simulink model "tanksReal"  (R2023a)
settings: Solver=VariableStepAuto  StartTime=0.0  StopTime=150  RelTol=1e-3
values from neighbouring files (symbols this model uses):
  a1 = 0.145    [main.m]
  a2 = 0.150    (= 0.15)    [main.m]
  A_a = 35    [main.m]
  fh = [3 4 5 6 7 8 9 10 11 12 13 14 15]    [main.m]
  fq = [17.75 21.65 23.76 27.55 30.01 31.98 33.88 38.18 46.28 49.88]    [main.m]
  fu = [0.5 1 1.5 2 2.5 3 3.5 5 8 10]    [main.m]
  fv = [0.909 1.685 2.475 3.255 4.055 4.804 5.573 6.332 7.121 7.847 8.617 9.405 10.18]    [main.m]
  h0 = 3.2    [main.m]
  Ts = 0.05    [main.m]
settings Model: Creator=vickay-0  LastModifiedBy=vickay-0

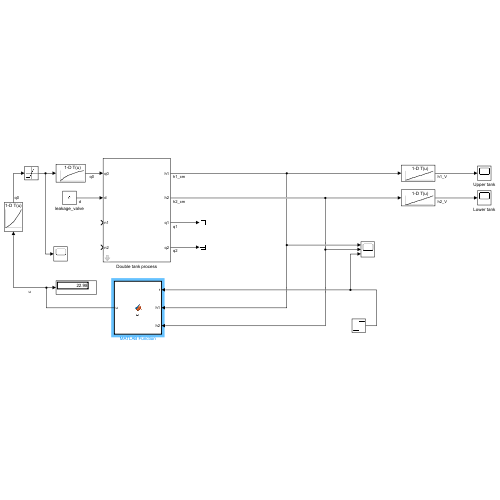
[thumbnail: Simulink's stored preview of the top-level diagram]
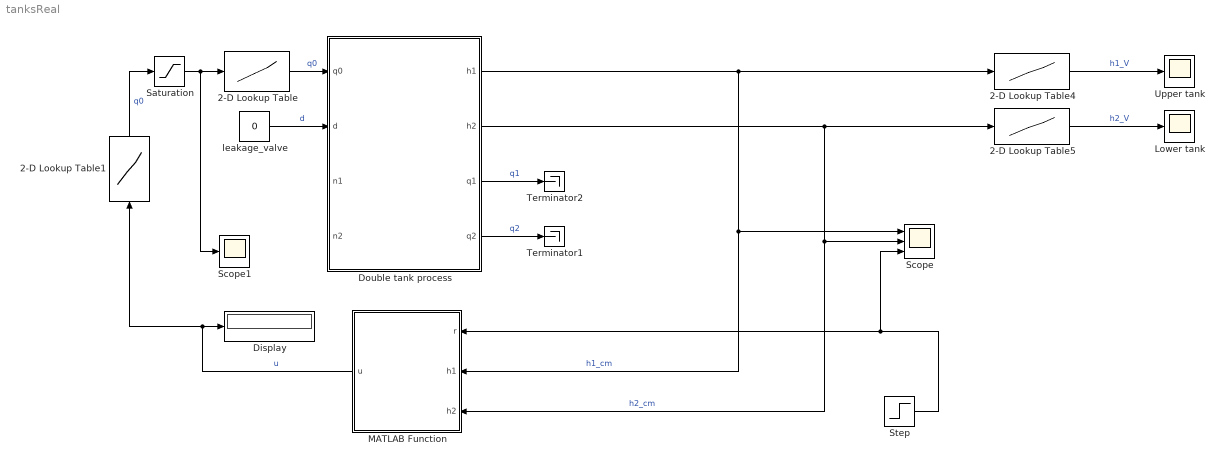
== system tanksReal ==
  2-D Lookup Table : Lookup_n-D  NumberOfTableDimensions=1  BreakpointsForDimension1=x  BreakpointsForDimension2=[1:3]  Table=y  RndMeth=Simplest  mask{x=fu, y=fq}
      mask prompts: x "Values on x-axis"; y "Values on y-axis"
  2-D Lookup Table1 : Lookup_n-D  NumberOfTableDimensions=1  BreakpointsForDimension1=x  BreakpointsForDimension2=[1:3]  Table=y  RndMeth=Simplest  mask{x=fq, y=fu}
      mask prompts: x "Values on x-axis"; y "Values on y-axis"
  2-D Lookup Table4 : Lookup_n-D  NumberOfTableDimensions=1  BreakpointsForDimension1=x  BreakpointsForDimension2=[1:3]  Table=y  RndMeth=Simplest  mask{x=fh, y=fv}
      mask prompts: x "Values on x-axis"; y "Values on y-axis"
  2-D Lookup Table5 : Lookup_n-D  NumberOfTableDimensions=1  BreakpointsForDimension1=x  BreakpointsForDimension2=[1:3]  Table=y  RndMeth=Simplest  mask{x=fh, y=fv}
      mask prompts: x "Values on x-axis"; y "Values on y-axis"
  Display : Display
  Double tank process : Subsystem  mask{At=A_a, Ao=a1, hmax=15.5}
      mask prompts: At "Tank area (cm^2)"; Ao "Opening area (cm^2)"; hmax "Tank height (cm)"
      mask help: Double tank process parameters
  Lower tank : Scope
  MATLAB Function : MATLAB Function  TreatAsAtomicUnit=on  SystemSampleTime=Ts
  Saturation : Saturate  UpperLimit=10  LowerLimit=0
  Scope : Scope  NumInputPorts=3
  Scope1 : Scope
  Step : Step  Time=50  Before=5  After=8  SampleTime=0
  Terminator1 : Terminator
  Terminator2 : Terminator
  Upper tank : Scope
  leakage_valve : Constant  Value=0
  wires:
  2-D Lookup Table5/1 -> Lower tank/1  "h2_V"
  Double tank process/3(q1) -> Terminator2/1  "q1"
  2-D Lookup Table/1 -> Double tank process/1(q0)  "q0"
  2-D Lookup Table4/1 -> Upper tank/1  "h1_V"
  MATLAB Function/1(u) -> Display/1, 2-D Lookup Table1/1  "u"
  Double tank process/4(q2) -> Terminator1/1  "q2"
  leakage_valve/1 -> Double tank process/2(d)  "d"
  Double tank process/2(h2) -> MATLAB Function/3(h2), Scope/2, 2-D Lookup Table5/1  "h2_cm"
  Double tank process/1(h1) -> Scope/1, MATLAB Function/2(h1), 2-D Lookup Table4/1  "h1_cm"
  Step/1 -> Scope/3, MATLAB Function/1(r)
  2-D Lookup Table1/1 -> Saturation/1  "q0"
  Saturation/1 -> Scope1/1, 2-D Lookup Table/1

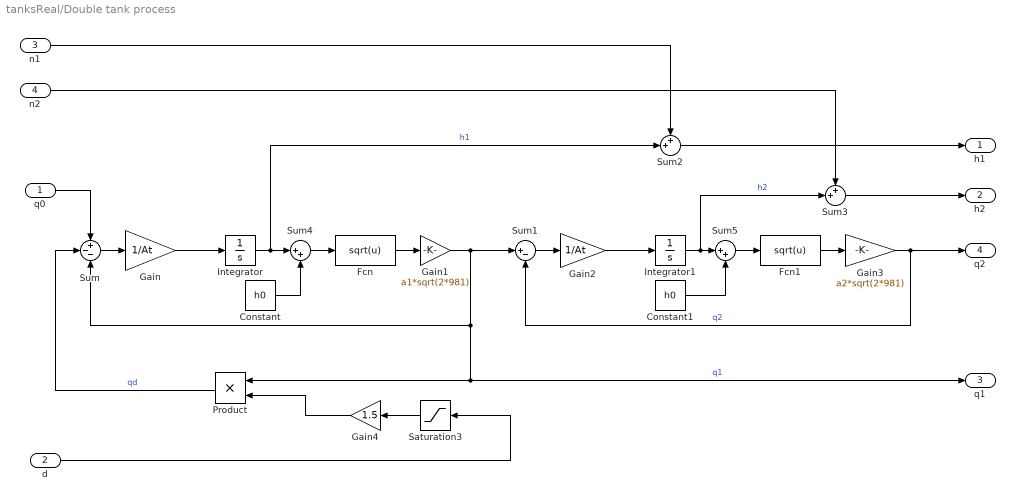
== system tanksReal/Double tank process ==
  q0 : Inport
  d : Inport  Port=2
  n1 : Inport  Port=3
  n2 : Inport  Port=4
  Constant : Constant  Value=h0
  Constant1 : Constant  Value=h0
  Fcn : Fcn  Expr=sqrt(u)
  Fcn1 : Fcn  Expr=sqrt(u)
  Gain : Gain  Gain=1/At
  Gain1 : Gain  Gain=a1*sqrt(2*981)
  Gain2 : Gain  Gain=1/At
  Gain3 : Gain  Gain=a2*sqrt(2*981)
  Gain4 : Gain  Gain=1.5
  Integrator : Integrator  LimitOutput=on  UpperSaturationLimit=hmax  LowerSaturationLimit=0
  Integrator1 : Integrator  LimitOutput=on  UpperSaturationLimit=hmax  LowerSaturationLimit=0
  Product : Product  RndMeth=Zero
  Saturation3 : Saturate  UpperLimit=1  LowerLimit=0
  Sum : Sum  Inputs=+--
  Sum1 : Sum  Inputs=|+-
  Sum2 : Sum  Inputs=++|
  Sum3 : Sum  Inputs=++|
  Sum4 : Sum  Inputs=|++
  Sum5 : Sum  Inputs=|++
  h1 : Outport  VectorParamsAs1DForOutWhenUnconnected=off
  h2 : Outport  Port=2  VectorParamsAs1DForOutWhenUnconnected=off
  q1 : Outport  Port=3  VectorParamsAs1DForOutWhenUnconnected=off
  q2 : Outport  Port=4  VectorParamsAs1DForOutWhenUnconnected=off
  wires:
  Sum/1 -> Gain/1
  Gain/1 -> Integrator/1
  Fcn/1 -> Gain1/1
  Gain1/1 -> Sum1/1, Product/1, q1/1, Sum/3  "q1"
  Sum1/1 -> Gain2/1
  Gain2/1 -> Integrator1/1
  Fcn1/1 -> Gain3/1
  Gain3/1 -> Sum1/2, q2/1  "q2"
  q0/1 -> Sum/1
  Integrator/1 -> Sum4/1, Sum2/2  "h1"
  Product/1 -> Sum/2  "qd"
  d/1 -> Saturation3/1
  Integrator1/1 -> Sum5/1, Sum3/2  "h2"
  Saturation3/1 -> Gain4/1
  Gain4/1 -> Product/2
  Sum2/1 -> h1/1
  n1/1 -> Sum2/1
  Sum3/1 -> h2/1
  n2/1 -> Sum3/1
  Sum4/1 -> Fcn/1
  Constant/1 -> Sum4/2
  Sum5/1 -> Fcn1/1
  Constant1/1 -> Sum5/2

== matlab function tanksReal/MATLAB Function ==
  data: r input; h1 input; h2 input; u output
function u  = fcn(r,h1,h2)

A = 35;   % Tank cross section
a1 = 0.145;   % Outlet cross section
a2 = 0.155;
g = 981;    % Gravity
h0 = 3.2; 

xi1 = h2;
xi2 = (sqrt(2)*a1*sqrt(g*(h0 + h1)))/A - (sqrt(2)*a2*sqrt(g*(h0 + h2)))/A;
%xi3 = (a1^2*g)/A^2 + (a2^2*g)/A^2 - (a1*a2*g*sqrt(g*h0 + g*h1))/(A^2*sqrt(g*h0 + g*h2)) - (sqrt(2)*a1*g*u_bar)/(2*A*sqrt(g*h0 + g*h1));

alfa =- (a1^2*g)/A^2 - (sqrt( (2))*a2*g*((sqrt( (2))*a1*sqrt(g*(h0 + h1)))/A - (sqrt( (2))*a2*sqrt(g*(h0 + h2)))/A))/(2*A*sqrt(g*(h0 + h2)));
beta = (sqrt( (2))*a1*g)/(2*A^2*sqrt(g*(h0 + h1)));
p1= -0.1;
p2=-2;
L = [ (-p1*-p2)  ,-(p1+p2)]';
Lr = (-p1*-p2);

u = (Lr*r - alfa + [-xi1 -xi2]*L)/beta;

end
